simulink model "version5"  (R2018b)
settings: Solver=FixedStepAuto  StartTime=0.0  StopTime=1  FixedStep=0.0005  RelTol=1e-3  EnableMultiTasking=on
model workspace (MAT data in the model file):
  APPS_1_X = [526 863 1200 1537 1837 2212 2310]
  APPS_2_X = [0 342 684 1026 1368 1710 1805]
  APPS_Y = [100 80 60 40 20 0 0]
  Motor_Temp = [0 25 50 75 85 100 115 125 150 175 200 225 ... (13 elements, 1x13)]
  duty_time = [0 1000 5000 6500 7500 9000 10000 10000 10000 10000 10000 10000 ... (13 elements, 1x13)]
undefined symbols (not defined in the file): I_AN06_5V, I_AN08_5V, I_AN09_5V, I_HALL1, I_SW11_H, O_PWM1_LS0A7, O_PWM2_LS0A7, O_SW01_LS0A4
libraries: ec5744lib x55, simulink x28, canmsglib x12, fuzblock x2
(part 3 of 3)

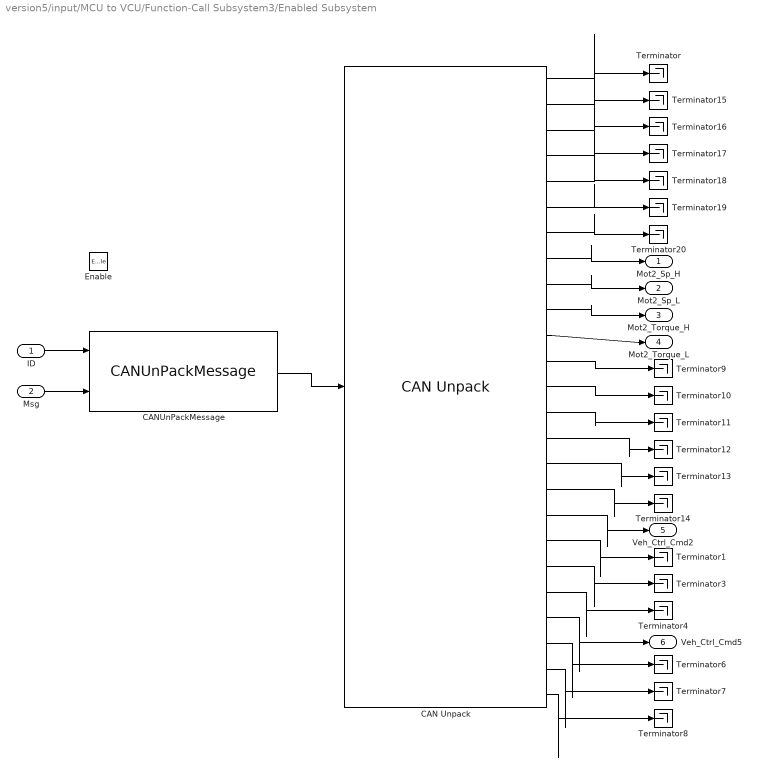
== system version5/input/MCU to VCU/Function-Call Subsystem3/Enabled Subsystem ==
  ID : Inport
  Msg : Inport  Port=2
  Enable : EnablePort
  CAN Unpack : canmsglib/CAN Unpack  CANdbFile=C:\WH\MC.dbc  MsgList=MCU2toVCU1_Ctrl  MsgName=MCU2toVCU1_Ctrl  MsgIDType=Extended (29-bit identifier)  MsgIdentifier=213000687  MsgLength=8  SignalInfo=Alarm_Reserved_Bit$50$1$1$2$1$0$1$0$0$1$#Bus_Over_Voltage$44$1$1$2$1$0$1$0$0$1$#Bus_Under_Voltag$46$1$1$2$1$0$1$0$0$1$#Combined_Alarm$56$2$1$2$1$0$1$0$0$3$#Control_Circuit_Anomaly$45$1$1$2$1$0$1$0$0$1$#Controller_Temp_Ala$48$1$1$2$1$0$1$0$0$1$#Ctrl_Rd$40$1$1$2$1$0$1$0$0$1$#Mot2_Sp_H$0$8$1$2$1$0$5.000000e-01$-10000$-10000$-9.872500e+03$#Mot2_Sp_L$8$8$1$2$1$0$5.000000e-01$-10000$-10000$-9.872500e+03$#Mot2_Torque_H$16$8$1$2$1$0$1$0$0$255$#Mot2_Torque_L$24$8$1$2$1$0$1$0$0$255$#Motor_Temp_Ala$49$1$1$2$1$0$1$0$0$1$#Over_Current$43$1$1$2$1$0$1$0$0$1$#Power_Limit$47$1$1$2$1$0$1$0$0$1$#Precharge_Condition$41$1$1$2$1$0$1$0$0$1$#Rotatory_Sen$42$1$1$2$1$0$1$0$0$1$#Self_Check$55$1$1$2$1$0$1$0$0$1$#Veh_Ctrl_Cmd1$32$1$1$2$1$0$1$0$0$1$#Veh_Ctrl_Cmd2$33$1$1$2$1$0$1$0$0$1$#Veh_Ctrl_Cmd3$34$1$1$2$1$0$1$0$0$1$#Veh_Ctrl_Cmd4$35$1$1$2$1$0$1$0$0$1$#Veh_Ctrl_Cmd5$36$1$1$2$1$0$1$0$0$1$#Veh_Ctrl_Cmd6$37$1$1$2$1$0$1$0$0$1$#Veh_Ctrl_Cmd7$38$1$1$2$1$0$1$0$0$1$#Veh_Ctrl_Cmd8$39$1$1$2$1$0$1$0$0$1$#  NSignals=25  IDPort=off  TimestampPort=off  ErrorPort=off  RemotePort=off  LengthPort=off  StatusPort=off  StartBits=str2num('[int32(50);int32(44);int32(46);int32(56);int32(45);int32(48);int32(40);int32(0);int32(8);int32(16);int32(24);int32(49);int32(43);int32(47);int32(41);int32(42);int32(55);int32(32);int32(33);int32(34);int32(35);int32(36);int32(37);int32(38);int32(39)]')  SignalSizes=str2num('[int32(1);int32(1);int32(1);int32(2);int32(1);int32(1);int32(1);int32(8);int32(8);int32(8);int32(8);int32(1);int32(1);int32(1);int32(1);int32(1);int32(1);int32(1);int32(1);int32(1);int32(1);int32(1);int32(1);int32(1);int32(1)]')  ByteOrders=str2num('[int32(1);int32(1);int32(1);int32(1);int32(1);int32(1);int32(1);int32(1);int32(1);int32(1);int32(1);int32(1);int32(1);int32(1);int32(1);int32(1);int32(1);int32(1);int32(1);int32(1);int32(1);int32(1);int32(1);int32(1);int32(1)]')  DataTypes=str2num('[int32(2);int32(2);int32(2);int32(2);int32(2);int32(2);int32(2);int32(2);int32(2);int32(2);int32(2);int32(2);int32(2);int32(2);int32(2);int32(2);int32(2);int32(2);int32(2);int32(2);int32(2);int32(2);int32(2);int32(2);int32(2)]')  MultiplexTypes=str2num('[int32(1);int32(1);int32(1);int32(1);int32(1);int32(1);int32(1);int32(1);int32(1);int32(1);int32(1);int32(1);int32(1);int32(1);int32(1);int32(1);int32(1);int32(1);int32(1);int32(1);int32(1);int32(1);int32(1);int32(1);int32(1)]')  MultiplexValues=str2num('[double(0);double(0);double(0);double(0);double(0);double(0);double(0);double(0);double(0);double(0);double(0);double(0);double(0);double(0);double(0);double(0);double(0);double(0);double(0);double(0);double(0);double(0);double(0);double(0);double(0)]')  Factors=str2num('[double(1);double(1);double(1);double(1);double(1);double(1);double(1);double(5.000000e-01);double(5.000000e-01);double(1);double(1);double(1);double(1);double(1);double(1);double(1);double(1);double(1);double(1);double(1);double(1);double(1);double(1);double(1);double(1)]')  Offsets=str2num('[double(0);double(0);double(0);double(0);double(0);double(0);double(0);double(-10000);double(-10000);double(0);double(0);double(0);double(0);double(0);double(0);double(0);double(0);double(0);double(0);double(0);double(0);double(0);double(0);double(0);double(0)]')  Minimums=str2num('[double(0);double(0);double(0);double(0);double(0);double(0);double(0);double(-10000);double(-10000);double(0);double(0);double(0);double(0);double(0);double(0);double(0);double(0);double(0);double(0);double(0);double(0);double(0);double(0);double(0);double(0)]')  Maximums=str2num('[double(1);double(1);double(1);double(3);double(1);double(1);double(1);double(-9.872500e+03);double(-9.872500e+03);double(255);double(255);double(1);double(1);double(1);double(1);double(1);double(1);double(1);double(1);double(1);double(1);double(1);double(1);double(1);double(1)]')  ApplyMinMax=off
      settings: SourceProductName=Simulink Real-Time  SourceProductBaseCode=XP  DataFormat=CANdb specified signals
  CANUnPackMessage : ec5744lib/RapidECU_U3/04CANCommunication/CANUnPackMessage  datalength=8  canmessagetype=Standard(11-bit ID)  sampletime=-1
      settings: SourceProductName=ECUCoder for MPC5744
  Terminator{,1,3..4,6..20} (19 alike) : Terminator
  Mot2_Sp_H : Outport
  Mot2_Sp_L : Outport  Port=2
  Mot2_Torque_H : Outport  Port=3
  Mot2_Torque_L : Outport  Port=4
  Veh_Ctrl_Cmd2 : Outport  Port=5
  Veh_Ctrl_Cmd5 : Outport  Port=6
  wires:
  Msg/1 -> CANUnPackMessage/2
  CANUnPackMessage/1 -> CAN Unpack/1
  ID/1 -> CANUnPackMessage/1
  CAN Unpack/8 -> Mot2_Sp_H/1
  CAN Unpack/9 -> Mot2_Sp_L/1
  CAN Unpack/11 -> Mot2_Torque_L/1
  CAN Unpack/10 -> Mot2_Torque_H/1
  CAN Unpack/18 -> Veh_Ctrl_Cmd2/1
  CAN Unpack/19 -> Terminator1/1
  CAN Unpack/20 -> Terminator3/1
  CAN Unpack/21 -> Terminator4/1
  CAN Unpack/22 -> Veh_Ctrl_Cmd5/1
  CAN Unpack/23 -> Terminator6/1
  CAN Unpack/24 -> Terminator7/1
  CAN Unpack/25 -> Terminator8/1
  CAN Unpack/12 -> Terminator9/1
  CAN Unpack/13 -> Terminator10/1
  CAN Unpack/14 -> Terminator11/1
  CAN Unpack/15 -> Terminator12/1
  CAN Unpack/16 -> Terminator13/1
  CAN Unpack/17 -> Terminator14/1
  CAN Unpack/4 -> Terminator17/1
  CAN Unpack/3 -> Terminator16/1
  CAN Unpack/2 -> Terminator15/1
  CAN Unpack/1 -> Terminator/1
  CAN Unpack/5 -> Terminator18/1
  CAN Unpack/6 -> Terminator19/1
  CAN Unpack/7 -> Terminator20/1

== system version5/input/MCUtoVCU/Function-Call Subsystem4/Enabled Subsystem ==
  ID : Inport
  Msg : Inport  Port=2
  Enable : EnablePort
  CAN Unpack : canmsglib/CAN Unpack  CANdbFile=C:\WH\MC.dbc  MsgList=MCU1toVCU2_Tp_Btv  MsgName=MCU1toVCU2_Tp_Btv  MsgIDType=Extended (29-bit identifier)  MsgIdentifier=218089455  MsgLength=8  SignalInfo=AC_Vaild_Value$48$16$1$2$1$0$1.000000e-01$-1600$-1600$4.953500e+03$#Controller_Temp1$0$8$1$2$1$0$1$-50$-50$200$#DC_Bus_Current1$32$16$1$2$1$0$1.000000e-01$-1600$-1600$4.953500e+03$#DC_Bus_Voltage$16$16$1$2$1$0$1.000000e-01$0$0$6.553500e+03$#Motor_Temp1$8$8$1$2$1$0$1$-50$-50$205$#  NSignals=5  IDPort=off  TimestampPort=off  ErrorPort=off  RemotePort=off  LengthPort=off  StatusPort=off  StartBits=str2num('[int32(48);int32(0);int32(32);int32(16);int32(8)]')  SignalSizes=str2num('[int32(16);int32(8);int32(16);int32(16);int32(8)]')  ByteOrders=str2num('[int32(1);int32(1);int32(1);int32(1);int32(1)]')  DataTypes=str2num('[int32(2);int32(2);int32(2);int32(2);int32(2)]')  MultiplexTypes=str2num('[int32(1);int32(1);int32(1);int32(1);int32(1)]')  MultiplexValues=str2num('[double(0);double(0);double(0);double(0);double(0)]')  Factors=str2num('[double(1.000000e-01);double(1);double(1.000000e-01);double(1.000000e-01);double(1)]')  Offsets=str2num('[double(-1600);double(-50);double(-1600);double(0);double(-50)]')  Minimums=str2num('[double(-1600);double(-50);double(-1600);double(0);double(-50)]')  Maximums=str2num('[double(4.953500e+03);double(200);double(4.953500e+03);double(6.553500e+03);double(205)]')  ApplyMinMax=off
      settings: SourceProductName=Simulink Real-Time  SourceProductBaseCode=XP  DataFormat=CANdb specified signals
  CANUnPackMessage : ec5744lib/RapidECU_U3/04CANCommunication/CANUnPackMessage  datalength=8  canmessagetype=Standard(11-bit ID)  sampletime=-1
      settings: SourceProductName=ECUCoder for MPC5744
  Terminator1 : Terminator
  Terminator18 : Terminator
  Terminator20 : Terminator
  MCU_Temp1 : Outport
  Motor_Temp1 : Outport  Port=2
  wires:
  Msg/1 -> CANUnPackMessage/2
  CANUnPackMessage/1 -> CAN Unpack/1
  ID/1 -> CANUnPackMessage/1
  CAN Unpack/2 -> MCU_Temp1/1
  CAN Unpack/5 -> Motor_Temp1/1
  CAN Unpack/4 -> Terminator20/1
  CAN Unpack/1 -> Terminator18/1
  CAN Unpack/3 -> Terminator1/1

== system version5/input/MCUtoVCU/Function-Call Subsystem5/Enabled Subsystem ==
  ID : Inport
  Msg : Inport  Port=2
  Enable : EnablePort
  CAN Unpack : canmsglib/CAN Unpack  CANdbFile=C:\WH\MC.dbc  MsgList=MCU2toVCU2_Tp_Btv  MsgName=MCU2toVCU2_Tp_Btv  MsgIDType=Extended (29-bit identifier)  MsgIdentifier=213066223  MsgLength=8  SignalInfo=AC_Vaild_Value$48$16$1$2$1$0$1.000000e-01$-1600$-1600$4.953500e+03$#Controller_Temp2$0$8$1$2$1$0$1$-50$-50$200$#DC_Bus_Current2$32$16$1$2$1$0$1.000000e-01$-1600$-1600$4.953500e+03$#DC_Bus_Voltage$16$16$1$2$1$0$1.000000e-01$0$0$6.553500e+03$#Motor_Temp2$8$8$1$2$1$0$1$-50$-50$200$#  NSignals=5  IDPort=off  TimestampPort=off  ErrorPort=off  RemotePort=off  LengthPort=off  StatusPort=off  StartBits=str2num('[int32(48);int32(0);int32(32);int32(16);int32(8)]')  SignalSizes=str2num('[int32(16);int32(8);int32(16);int32(16);int32(8)]')  ByteOrders=str2num('[int32(1);int32(1);int32(1);int32(1);int32(1)]')  DataTypes=str2num('[int32(2);int32(2);int32(2);int32(2);int32(2)]')  MultiplexTypes=str2num('[int32(1);int32(1);int32(1);int32(1);int32(1)]')  MultiplexValues=str2num('[double(0);double(0);double(0);double(0);double(0)]')  Factors=str2num('[double(1.000000e-01);double(1);double(1.000000e-01);double(1.000000e-01);double(1)]')  Offsets=str2num('[double(-1600);double(-50);double(-1600);double(0);double(-50)]')  Minimums=str2num('[double(-1600);double(-50);double(-1600);double(0);double(-50)]')  Maximums=str2num('[double(4.953500e+03);double(200);double(4.953500e+03);double(6.553500e+03);double(200)]')  ApplyMinMax=off
      settings: SourceProductName=Simulink Real-Time  SourceProductBaseCode=XP  DataFormat=CANdb specified signals
  CANUnPackMessage : ec5744lib/RapidECU_U3/04CANCommunication/CANUnPackMessage  datalength=8  canmessagetype=Standard(11-bit ID)  sampletime=-1
      settings: SourceProductName=ECUCoder for MPC5744
  Terminator11 : Terminator
  Terminator12 : Terminator
  Terminator20 : Terminator
  MCU_Temp2 : Outport
  Motor_Temp2 : Outport  Port=2
  wires:
  Msg/1 -> CANUnPackMessage/2
  CANUnPackMessage/1 -> CAN Unpack/1
  ID/1 -> CANUnPackMessage/1
  CAN Unpack/5 -> Motor_Temp2/1
  CAN Unpack/2 -> MCU_Temp2/1
  CAN Unpack/4 -> Terminator12/1
  CAN Unpack/3 -> Terminator11/1
  CAN Unpack/1 -> Terminator20/1

== stateflow chart version5/control/start/Chart1 ==
  state B
    en:
    O_SwitchH_1 = 1;
    O_SwitchL_2 = 0;
    Veh_Ctrl_Cmd2=1;
    Veh_Ctrl_Cmd5=0;
    READY=0;
  note: 加速踏板标志位1    踏板未踩动，
      | 				 0    踏板踩动
      | KEY待驶按钮   1    按下点火
      | 制动踏板标志位1    制动抱死
      |                          0    松开踏板
  state A
    en:
    O_SwitchL_2 =1;
    O_SwitchH_1 = 1;
    Veh_Ctrl_Cmd2=0;
    Veh_Ctrl_Cmd5=1;
    READY=0;
  state C
    en:
    O_SwitchH_1 = 0;
    O_SwitchL_2 = 0;
    Veh_Ctrl_Cmd2=1;
    Veh_Ctrl_Cmd5=0;
    READY=1;
  A -> B : [acc==1&KEY~=0&Brake_F==1]
  B -> C : after (3,sec)
  (default) -> A
  C -> A : [acc==0&KEY==0&Brake_F==0]
  data: KEY input; acc input; Brake_F input; O_SwitchH_1 output; O_SwitchL_2 output; Veh_Ctrl_Cmd2 output; Veh_Ctrl_Cmd5 output; READY output

== matlab function version5/control/APS_Ctrl/clock/计时计数/MATLAB Function ==
  data: Bukekao output; u input; y output; continuous_num input; old_u input
function [Bukekao,y] = fcn(u,continuous_num,old_u)
%
%
%出现踏板不可靠
if(u==1)
    y = 1+old_u;        %输出的不可靠次数y = 累计次数 + 1；
else
    y=0;                %输出可靠后清除不可靠信号
end
if(y>continuous_num)    %当不可靠次数y > 设定的阈值次数
    Bukekao=1;          %不可靠输出 1 
else
    Bukekao=0;          %否则不可靠输出 0
end
if(y>100)
    y = 100;
end

== stateflow chart version5/control/APS_Ctrl/Aps_Reliable1 ==
  (default) -> (junction 14) : /* 加速踏板信号可靠的检测 */
  (junction 14) -> (junction 15) : [APS1_OP > 100 || APS2_OP > 100]
  (junction 15) -> (junction 17) : {Pedal_WrongState = 1;}
  (junction 17) -> (junction 16)
  (junction 16) -> (junction 18)
  data: APS1_OP input uint8; APS2_OP input uint8; Pedal_WrongState output boolean

== stateflow chart version5/control/Chart1 ==
  state Cal1
    du:
    SpeedL = 0;
    SpeedR = 0;
  state Cal
    du:
    SpeedL = 1/Gear_NumL*2*3.14*0.2286*3.6;
    SpeedR = 1/Gear_NumR*2*3.14*0.2286*3.6;
  (default) -> Cal1
  Cal1 -> Cal : [Gear_NumL && Gear_NumR !=0]
  Cal -> Cal1 : [Gear_NumL && Gear_NumR ==0]
  data: Gear_NumL input; SpeedL output double; Gear_NumR input; SpeedR output double
